simulink model "Network_Standalone"  (R2018b)
settings: Solver=VariableStepAuto  StartTime=0.0  StopTime=10  RelTol=1e-3
undefined symbols (not defined in the file): B, Kd, Ts
libraries: simulink x9
settings Model: Creator=oscar  LastModifiedBy=oscar

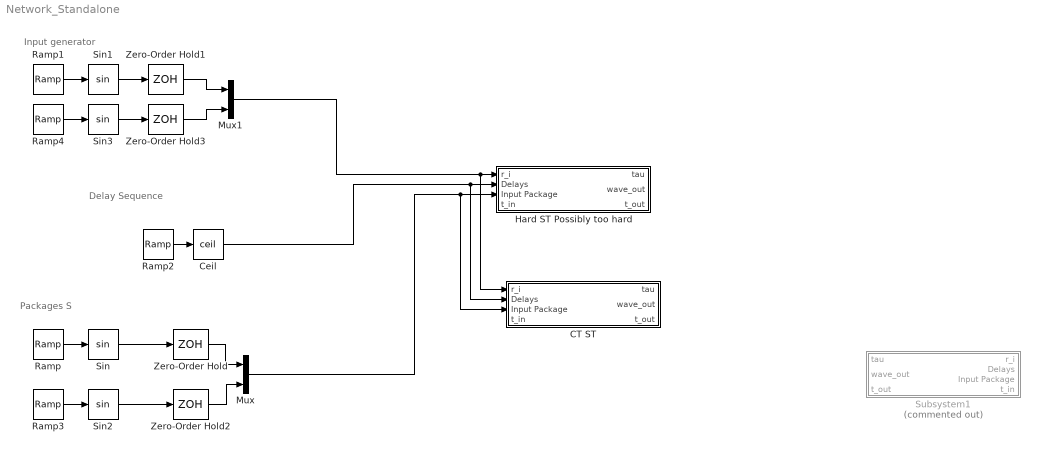
== system Network_Standalone ==
  note: Input generator
  note: Packages S
  note: Delay Sequence
  CT ST : Subsystem
  Ceil : Rounding  Operator=ceil
  Hard ST Possibly too hard : Subsystem
  Mux : Mux  Inputs=2
  Mux1 : Mux  Inputs=2
  Ramp : simulink/Sources/Ramp  slope=1  start=0  InitialOutput=0
  Ramp1 : simulink/Sources/Ramp  slope=1  start=0  InitialOutput=0
  Ramp2 : simulink/Sources/Ramp  slope=0.3/Ts  start=0  InitialOutput=5
  Ramp3 : simulink/Sources/Ramp  slope=0.9  start=1  InitialOutput=0
  Ramp4 : simulink/Sources/Ramp  slope=0.5  start=0  InitialOutput=0
  Sin{,1..3} (4 alike) : Trigonometry
  Subsystem1 : Subsystem  Commented=on
  Zero-Order Hold{,1..3} (4 alike) : ZeroOrderHold  SampleTime=Ts
  wires:
  Ramp/1 -> Sin/1
  Zero-Order Hold/1 -> Mux/1
  Sin/1 -> Zero-Order Hold/1
  Ramp2/1 -> Ceil/1
  Ceil/1 -> CT ST/2(Delays), Hard ST Possibly too hard/2(Delays)
  Zero-Order Hold1/1 -> Mux1/1
  Ramp1/1 -> Sin1/1
  Sin1/1 -> Zero-Order Hold1/1
  Ramp3/1 -> Sin2/1
  Sin2/1 -> Zero-Order Hold2/1
  Mux/1 -> CT ST/3(Input Package), Hard ST Possibly too hard/3(Input Package)
  Zero-Order Hold2/1 -> Mux/2
  Zero-Order Hold3/1 -> Mux1/2
  Mux1/1 -> CT ST/1(r_i), Hard ST Possibly too hard/1(r_i)
  Ramp4/1 -> Sin3/1
  Sin3/1 -> Zero-Order Hold3/1

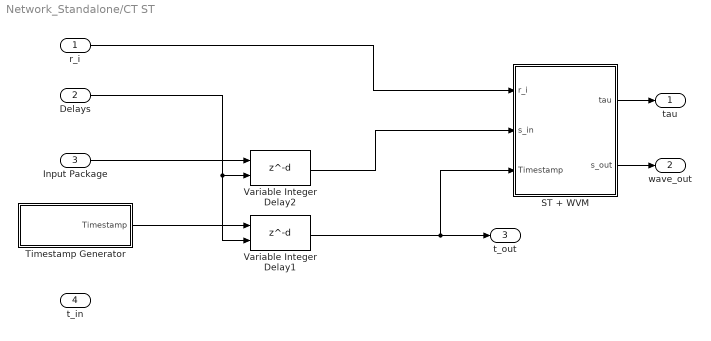
== system Network_Standalone/CT ST ==
  r_i : Inport
  Delays : Inport  Port=2
  Input Package : Inport  Port=3
  t_in : Inport  Port=4
  ST + WVM : Subsystem  TreatAsAtomicUnit=on
  Timestamp Generator : Subsystem
  Variable Integer Delay1 : Delay  DelayLengthSource=Input port  PreventDirectFeedthrough=on  SampleTime=Ts
      settings: InputPortMap=u0,p1
  Variable Integer Delay2 : Delay  DelayLengthSource=Input port  PreventDirectFeedthrough=on  SampleTime=Ts
      settings: InputPortMap=u0,p1
  tau : Outport
  wave_out : Outport  Port=2
  t_out : Outport  Port=3
  wires:
  Input Package/1 -> Variable Integer Delay2/1
  Variable Integer Delay2/1 -> ST + WVM/2(s_in)
  Delays/1 -> Variable Integer Delay1/2, Variable Integer Delay2/2
  Timestamp Generator/1(Timestamp) -> Variable Integer Delay1/1
  r_i/1 -> ST + WVM/1(r_i)
  ST + WVM/1(tau) -> tau/1
  ST + WVM/2(s_out) -> wave_out/1
  Variable Integer Delay1/1 -> ST + WVM/3(Timestamp), t_out/1

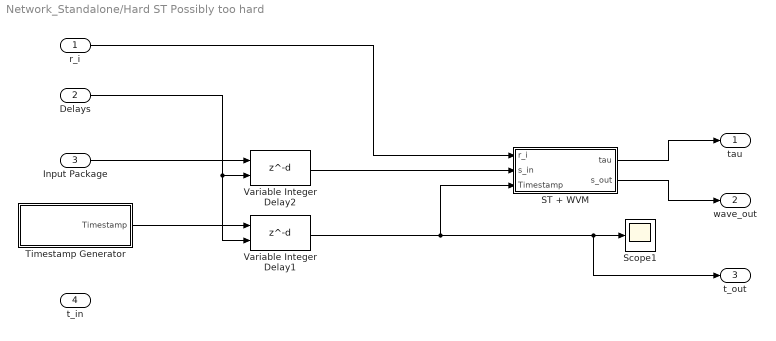
== system Network_Standalone/Hard ST Possibly too hard ==
  r_i : Inport
  Delays : Inport  Port=2
  Input Package : Inport  Port=3
  t_in : Inport  Port=4
  ST + WVM : Subsystem  TreatAsAtomicUnit=on
  Scope1 : Scope
  Timestamp Generator : Subsystem
  Variable Integer Delay1 : Delay  DelayLengthSource=Input port  PreventDirectFeedthrough=on  SampleTime=Ts
      settings: InputPortMap=u0,p1
  Variable Integer Delay2 : Delay  DelayLengthSource=Input port  PreventDirectFeedthrough=on  SampleTime=Ts
      settings: InputPortMap=u0,p1
  tau : Outport
  wave_out : Outport  Port=2
  t_out : Outport  Port=3
  wires:
  Input Package/1 -> Variable Integer Delay2/1
  Variable Integer Delay2/1 -> ST + WVM/2(s_in)
  Delays/1 -> Variable Integer Delay1/2, Variable Integer Delay2/2
  Timestamp Generator/1(Timestamp) -> Variable Integer Delay1/1
  r_i/1 -> ST + WVM/1(r_i)
  ST + WVM/1(tau) -> tau/1
  ST + WVM/2(s_out) -> wave_out/1
  Variable Integer Delay1/1 -> ST + WVM/3(Timestamp), t_out/1, Scope1/1

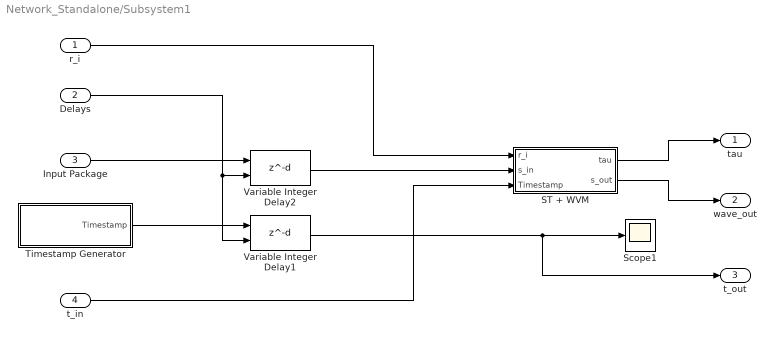
== system Network_Standalone/Subsystem1 ==
  r_i : Inport
  Delays : Inport  Port=2
  Input Package : Inport  Port=3
  t_in : Inport  Port=4
  ST + WVM : Subsystem  TreatAsAtomicUnit=on
  Scope1 : Scope
  Timestamp Generator : Subsystem
  Variable Integer Delay1 : Delay  DelayLengthSource=Input port  PreventDirectFeedthrough=on  SampleTime=Ts
      settings: InputPortMap=u0,p1
  Variable Integer Delay2 : Delay  DelayLengthSource=Input port  PreventDirectFeedthrough=on  SampleTime=Ts
      settings: InputPortMap=u0,p1
  tau : Outport
  wave_out : Outport  Port=2
  t_out : Outport  Port=3
  wires:
  Input Package/1 -> Variable Integer Delay2/1
  Variable Integer Delay2/1 -> ST + WVM/2(s_in)
  Delays/1 -> Variable Integer Delay1/2, Variable Integer Delay2/2
  Timestamp Generator/1(Timestamp) -> Variable Integer Delay1/1
  Variable Integer Delay1/1 -> t_out/1, Scope1/1
  r_i/1 -> ST + WVM/1(r_i)
  ST + WVM/1(tau) -> tau/1
  ST + WVM/2(s_out) -> wave_out/1
  t_in/1 -> ST + WVM/3(Timestamp)

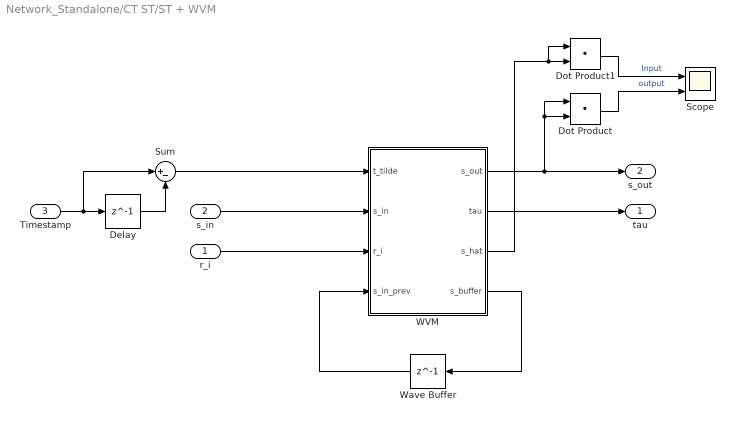
== system Network_Standalone/CT ST/ST + WVM ==
  r_i : Inport
  s_in : Inport  Port=2
  Timestamp : Inport  Port=3
  Delay : Delay  DelayLength=1  SampleTime=Ts
  Dot Product : DotProduct  InputSameDT=on  OutDataTypeStr=Inherit: Inherit via internal rule
  Dot Product1 : DotProduct  InputSameDT=on  OutDataTypeStr=Inherit: Inherit via internal rule
  Scope : Scope  NumInputPorts=2
  Sum : Sum  Inputs=|+-
  WVM : MATLAB Function  TreatAsAtomicUnit=on
  Wave Buffer : Delay  DelayLength=1  InitialCondition=[0;0]  SampleTime=Ts
  tau : Outport
  s_out : Outport  Port=2
  wires:
  Timestamp/1 -> Sum/1, Delay/1
  Delay/1 -> Sum/2
  WVM/2(tau) -> tau/1
  WVM/1(s_out) -> Dot Product/2, Dot Product/1, s_out/1
  WVM/4(s_buffer) -> Wave Buffer/1
  Wave Buffer/1 -> WVM/4(s_in_prev)
  Sum/1 -> WVM/1(t_tilde)
  s_in/1 -> WVM/2(s_in)
  r_i/1 -> WVM/3(r_i)
  WVM/3(s_hat) -> Dot Product1/1, Dot Product1/2
  Dot Product1/1 -> Scope/1  "Input"
  Dot Product/1 -> Scope/2  "output"

== system Network_Standalone/CT ST/Timestamp Generator ==
  note: Timestamp
  Ramp1 : simulink/Sources/Ramp  slope=1/Ts  start=0  InitialOutput=0
  Rounding Function : Rounding
  Timestamp : Outport
  wires:
  Rounding Function/1 -> Timestamp/1
  Ramp1/1 -> Rounding Function/1

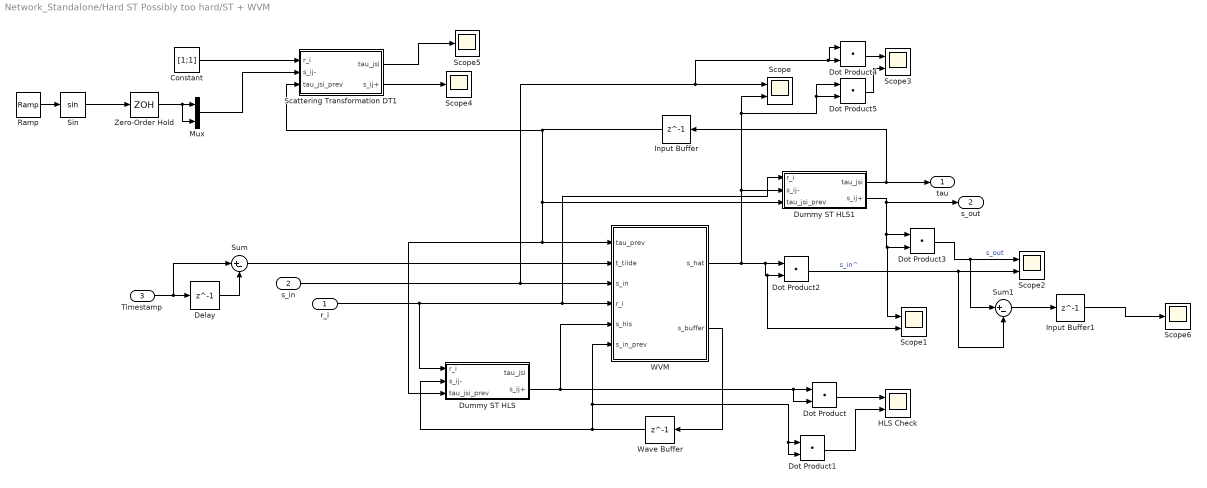
== system Network_Standalone/Hard ST Possibly too hard/ST + WVM ==
  r_i : Inport
  s_in : Inport  Port=2
  Timestamp : Inport  Port=3
  Constant : Constant  Value=[1;1]
  Delay : Delay  DelayLength=1  SampleTime=Ts
  Dot Product{,1..5} (6 alike) : DotProduct  InputSameDT=on  OutDataTypeStr=Inherit: Inherit via internal rule
  Dummy ST HLS : Subsystem
  Dummy ST HLS1 : Subsystem
  HLS Check : Scope  NumInputPorts=2
  Input Buffer : Delay  DelayLength=1  InitialCondition=[0;0]  SampleTime=Ts
  Input Buffer1 : Delay  DelayLength=1  InitialCondition=[0;0]  SampleTime=Ts
  Mux : Mux  Inputs=2
  Ramp : simulink/Sources/Ramp  slope=1  start=0  InitialOutput=0
  Scattering Transformation DT1 : Subsystem
  Scope{,1..3} (4 alike) : Scope  NumInputPorts=2
  Scope4 : Scope
  Scope5 : Scope
  Scope6 : Scope
  Sin : Trigonometry
  Sum : Sum  Inputs=|+-
  Sum1 : Sum  Inputs=|+-
  WVM : MATLAB Function  TreatAsAtomicUnit=on
  Wave Buffer : Delay  DelayLength=1  InitialCondition=[0;0]  SampleTime=Ts
  Zero-Order Hold : ZeroOrderHold  SampleTime=Ts
  tau : Outport
  s_out : Outport  Port=2
  wires:
  Timestamp/1 -> Sum/1, Delay/1
  Delay/1 -> Sum/2
  r_i/1 -> Dummy ST HLS1/1(r_i), WVM/4(r_i), Dummy ST HLS/1(r_i)
  Dummy ST HLS/2(s_ij+) -> Dot Product/2, Dot Product/1, WVM/5(s_hls)
  Dummy ST HLS1/1(tau_jsi) -> Input Buffer/1, tau/1
  Dummy ST HLS1/2(s_ij+) -> Dot Product3/1, Scope1/1, Dot Product3/2, s_out/1
  s_in/1 -> Dot Product4/1, Dot Product4/2, Scope/1, WVM/3(s_in)
  WVM/2(s_buffer) -> Wave Buffer/1
  Sum/1 -> WVM/2(t_tilde)
  Input Buffer/1 -> Scattering Transformation DT1/3(tau_jsi_prev), Dummy ST HLS1/3(tau_jsi_prev), WVM/1(tau_prev), Dummy ST HLS/3(tau_jsi_prev)
  WVM/1(s_hat) -> Scope1/2, Dot Product2/2, Dot Product2/1, Dummy ST HLS1/2(s_ij-), Dot Product5/2, Dot Product5/1, Scope/2
  Dot Product/1 -> HLS Check/1
  Wave Buffer/1 -> Dot Product1/2, Dot Product1/1, WVM/6(s_in_prev), Dummy ST HLS/2(s_ij-)
  Dot Product1/1 -> HLS Check/2
  Dot Product3/1 -> Sum1/1, Scope2/1  "s_out"
  Dot Product4/1 -> Scope3/1
  Dot Product5/1 -> Scope3/2
  Constant/1 -> Scattering Transformation DT1/1(r_i)
  Zero-Order Hold/1 -> Mux/2, Mux/1
  Sin/1 -> Zero-Order Hold/1
  Ramp/1 -> Sin/1
  Scattering Transformation DT1/2(s_ij+) -> Scope4/1
  Scattering Transformation DT1/1(tau_jsi) -> Scope5/1
  Mux/1 -> Scattering Transformation DT1/2(s_ij-)
  Dot Product2/1 -> Sum1/2, Scope2/2  "s_in^"
  Sum1/1 -> Input Buffer1/1
  Input Buffer1/1 -> Scope6/1

== system Network_Standalone/Hard ST Possibly too hard/Timestamp Generator ==
  note: Timestamp
  Ramp1 : simulink/Sources/Ramp  slope=1/Ts  start=0  InitialOutput=0
  Rounding Function : Rounding
  Timestamp : Outport
  wires:
  Rounding Function/1 -> Timestamp/1
  Ramp1/1 -> Rounding Function/1

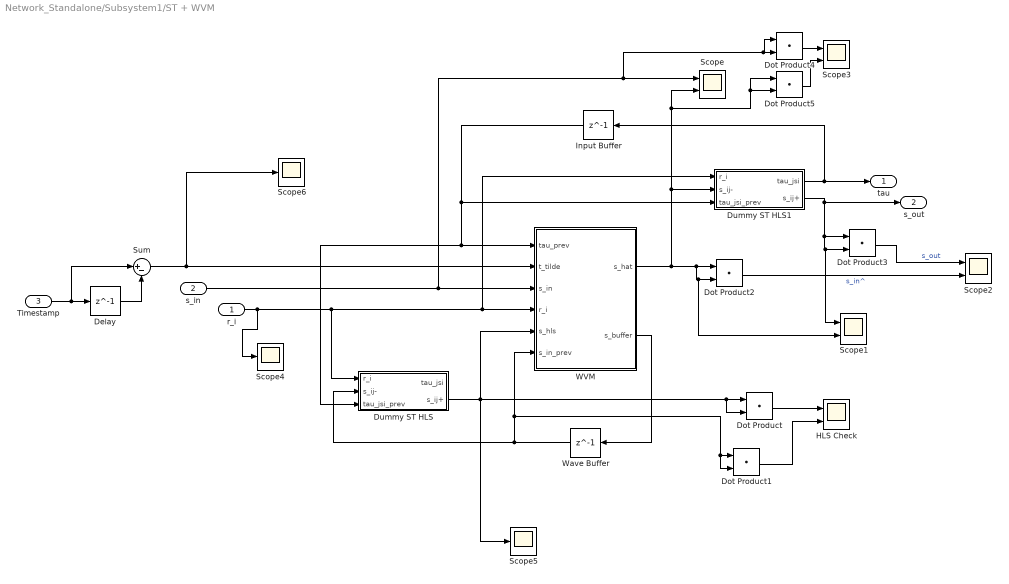
== system Network_Standalone/Subsystem1/ST + WVM ==
  r_i : Inport
  s_in : Inport  Port=2
  Timestamp : Inport  Port=3
  Delay : Delay  DelayLength=1  SampleTime=Ts
  Dot Product{,1..5} (6 alike) : DotProduct  InputSameDT=on  OutDataTypeStr=Inherit: Inherit via internal rule
  Dummy ST HLS : Subsystem
  Dummy ST HLS1 : Subsystem
  HLS Check : Scope  NumInputPorts=2
  Input Buffer : Delay  DelayLength=1  InitialCondition=[0;0]  SampleTime=Ts
  Scope{,1..3} (4 alike) : Scope  NumInputPorts=2
  Scope4 : Scope
  Scope5 : Scope
  Scope6 : Scope
  Sum : Sum  Inputs=|+-
  WVM : MATLAB Function  TreatAsAtomicUnit=on
  Wave Buffer : Delay  DelayLength=1  InitialCondition=[0;0]  SampleTime=Ts
  tau : Outport
  s_out : Outport  Port=2
  wires:
  Timestamp/1 -> Sum/1, Delay/1
  Delay/1 -> Sum/2
  r_i/1 -> Scope4/1, Dummy ST HLS1/1(r_i), WVM/4(r_i), Dummy ST HLS/1(r_i)
  Dummy ST HLS/2(s_ij+) -> Scope5/1, Dot Product/2, Dot Product/1, WVM/5(s_hls)
  Dummy ST HLS1/1(tau_jsi) -> Input Buffer/1, tau/1
  Dummy ST HLS1/2(s_ij+) -> Dot Product3/1, Scope1/1, Dot Product3/2, s_out/1
  s_in/1 -> Dot Product4/1, Dot Product4/2, Scope/1, WVM/3(s_in)
  WVM/2(s_buffer) -> Wave Buffer/1
  Sum/1 -> Scope6/1, WVM/2(t_tilde)
  Input Buffer/1 -> Dummy ST HLS1/3(tau_jsi_prev), WVM/1(tau_prev), Dummy ST HLS/3(tau_jsi_prev)
  WVM/1(s_hat) -> Scope1/2, Dot Product2/2, Dot Product2/1, Dummy ST HLS1/2(s_ij-), Dot Product5/2, Dot Product5/1, Scope/2
  Dot Product/1 -> HLS Check/1
  Wave Buffer/1 -> Dot Product1/2, Dot Product1/1, WVM/6(s_in_prev), Dummy ST HLS/2(s_ij-)
  Dot Product1/1 -> HLS Check/2
  Dot Product3/1 -> Scope2/1  "s_out"
  Dot Product4/1 -> Scope3/1
  Dot Product5/1 -> Scope3/2
  Dot Product2/1 -> Scope2/2  "s_in^"

== system Network_Standalone/Subsystem1/Timestamp Generator ==
  note: Timestamp
  Ramp1 : simulink/Sources/Ramp  slope=1/Ts  start=0  InitialOutput=0
  Rounding Function : Rounding
  Timestamp : Outport
  wires:
  Rounding Function/1 -> Timestamp/1
  Ramp1/1 -> Rounding Function/1

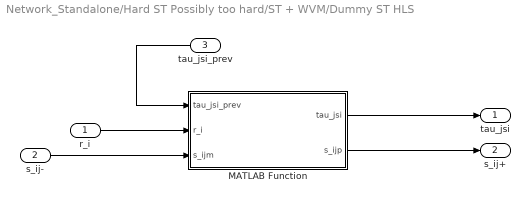
== system Network_Standalone/Hard ST Possibly too hard/ST + WVM/Dummy ST HLS ==
  r_i : Inport
  s_ij- : Inport  Port=2
  tau_jsi_prev : Inport  Port=3
  MATLAB Function : MATLAB Function  TreatAsAtomicUnit=on
  tau_jsi : Outport
  s_ij+ : Outport  Port=2
  wires:
  MATLAB Function/1(tau_jsi) -> tau_jsi/1
  tau_jsi_prev/1 -> MATLAB Function/1(tau_jsi_prev)
  r_i/1 -> MATLAB Function/2(r_i)
  s_ij-/1 -> MATLAB Function/3(s_ijm)
  MATLAB Function/2(s_ijp) -> s_ij+/1

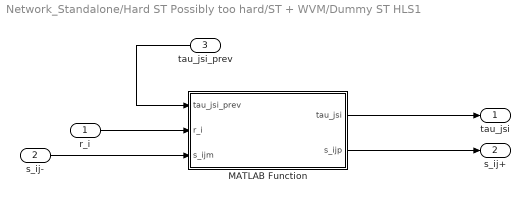
== system Network_Standalone/Hard ST Possibly too hard/ST + WVM/Dummy ST HLS1 ==
  r_i : Inport
  s_ij- : Inport  Port=2
  tau_jsi_prev : Inport  Port=3
  MATLAB Function : MATLAB Function  TreatAsAtomicUnit=on
  tau_jsi : Outport
  s_ij+ : Outport  Port=2
  wires:
  MATLAB Function/1(tau_jsi) -> tau_jsi/1
  tau_jsi_prev/1 -> MATLAB Function/1(tau_jsi_prev)
  r_i/1 -> MATLAB Function/2(r_i)
  s_ij-/1 -> MATLAB Function/3(s_ijm)
  MATLAB Function/2(s_ijp) -> s_ij+/1

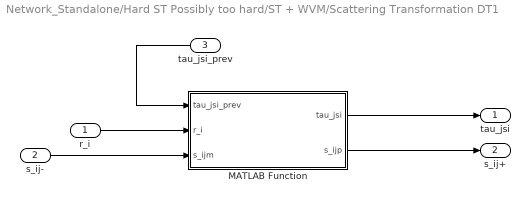
== system Network_Standalone/Hard ST Possibly too hard/ST + WVM/Scattering Transformation DT1 ==
  r_i : Inport
  s_ij- : Inport  Port=2
  tau_jsi_prev : Inport  Port=3
  MATLAB Function : MATLAB Function  TreatAsAtomicUnit=on
  tau_jsi : Outport
  s_ij+ : Outport  Port=2
  wires:
  MATLAB Function/1(tau_jsi) -> tau_jsi/1
  tau_jsi_prev/1 -> MATLAB Function/1(tau_jsi_prev)
  r_i/1 -> MATLAB Function/2(r_i)
  s_ij-/1 -> MATLAB Function/3(s_ijm)
  MATLAB Function/2(s_ijp) -> s_ij+/1

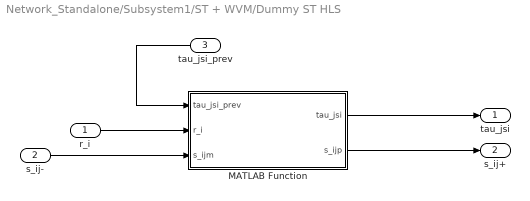
== system Network_Standalone/Subsystem1/ST + WVM/Dummy ST HLS ==
  r_i : Inport
  s_ij- : Inport  Port=2
  tau_jsi_prev : Inport  Port=3
  MATLAB Function : MATLAB Function  TreatAsAtomicUnit=on
  tau_jsi : Outport
  s_ij+ : Outport  Port=2
  wires:
  MATLAB Function/1(tau_jsi) -> tau_jsi/1
  tau_jsi_prev/1 -> MATLAB Function/1(tau_jsi_prev)
  r_i/1 -> MATLAB Function/2(r_i)
  s_ij-/1 -> MATLAB Function/3(s_ijm)
  MATLAB Function/2(s_ijp) -> s_ij+/1

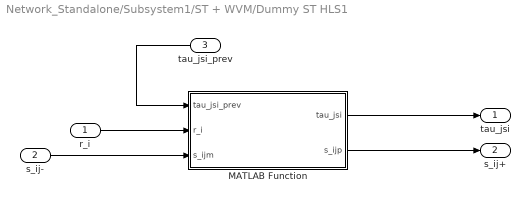
== system Network_Standalone/Subsystem1/ST + WVM/Dummy ST HLS1 ==
  r_i : Inport
  s_ij- : Inport  Port=2
  tau_jsi_prev : Inport  Port=3
  MATLAB Function : MATLAB Function  TreatAsAtomicUnit=on
  tau_jsi : Outport
  s_ij+ : Outport  Port=2
  wires:
  MATLAB Function/1(tau_jsi) -> tau_jsi/1
  tau_jsi_prev/1 -> MATLAB Function/1(tau_jsi_prev)
  r_i/1 -> MATLAB Function/2(r_i)
  s_ij-/1 -> MATLAB Function/3(s_ijm)
  MATLAB Function/2(s_ijp) -> s_ij+/1

== matlab function Network_Standalone/Hard ST Possibly too hard/ST + WVM/Scattering Transformation DT1/MATLAB Function ==
  data: tau_jsi_prev input; r_i input; tau_jsi output; s_ijm input; s_ijp output; B parameter; Kd parameter
function [tau_jsi, s_ijp] = STL(tau_jsi_prev,r_i, s_ijm, B, Kd)
    tau_jsi = zeros(2, 1);
    s_ijp = zeros(2, 1);
    
    r_js = (inv(B))^2*(-sqrt(2)*B*s_ijm - tau_jsi_prev);
    tau_jsi = Kd*(r_js - r_i);
    s_ijp = 1/sqrt(2)*inv(B)*(-tau_jsi + B^2*r_js);
end

== matlab function Network_Standalone/Hard ST Possibly too hard/ST + WVM/Dummy ST HLS1/MATLAB Function ==
  data: tau_jsi_prev input; r_i input; tau_jsi output; s_ijm input; s_ijp output; B parameter; Kd parameter
function [tau_jsi, s_ijp] = STL(tau_jsi_prev,r_i, s_ijm, B, Kd)
    tau_jsi = zeros(2, 1);
    s_ijp = zeros(2, 1);
    
    r_js = (inv(B))^2*(-sqrt(2)*B*s_ijm - tau_jsi_prev);
    tau_jsi = Kd*(r_js - r_i);
    s_ijp = 1/sqrt(2)*inv(B)*(-tau_jsi_prev + B^2*r_js);
end

== matlab function Network_Standalone/Hard ST Possibly too hard/ST + WVM/WVM ==
  data: tau_prev input; t_tilde input; s_in input; r_i input; s_hls input; s_in_prev input; s_hat output; s_buffer output
function [s_hat, s_buffer]  = fcn(tau_prev, t_tilde, s_in, r_i, s_hls, s_in_prev)
    s_hat = zeros(2, 1);
    s_buffer = zeros(2, 1);
    
    %% If 0 then no new data -> reconstruct!
    % If lower than 0, then the package is reordered and we reject the
    % package
    if(t_tilde <= 0)  
        % If HLS is passive apply HLS
        if(s_hls'*s_hls >= s_in_prev'*s_in_prev)
            s_hat = s_in_prev;
            
        % Otherwise apply the acceptable magnitude in that direction
        else
            s_hat = zeros(2,1);%sign(s_in_prev).*abs(s_hls)./sqrt(2);
            %s_hat = sign(s_in_prev) .* abs(1/sqrt(2)*r_i); % WVM Gain (Dit is nie netjes)
        end
        
        % Either way repeat the last value
        s_buffer = s_in_prev;
        
    %% If 1 then no weird shenanigans, data arrived on time
    %% If > 1 then the packages are reordered and we keep the last one
    else
        s_hat = s_in; % Use the received value
        s_buffer = s_in; % And store its value
    end    

end

== matlab function Network_Standalone/Hard ST Possibly too hard/ST + WVM/Dummy ST HLS/MATLAB Function ==
  data: tau_jsi_prev input; r_i input; tau_jsi output; s_ijm input; s_ijp output; B parameter; Kd parameter
function [tau_jsi, s_ijp] = STL(tau_jsi_prev,r_i, s_ijm, B, Kd)
    tau_jsi = zeros(2, 1);
    s_ijp = zeros(2, 1);
    
    r_js = (inv(B))^2*(-sqrt(2)*B*s_ijm - tau_jsi_prev);
    tau_jsi = Kd*(r_js - r_i);
    s_ijp = 1/sqrt(2)*inv(B)*(-tau_jsi_prev + B^2*r_js);
end

== matlab function Network_Standalone/Subsystem1/ST + WVM/Dummy ST HLS/MATLAB Function ==
  data: tau_jsi_prev input; r_i input; tau_jsi output; s_ijm input; s_ijp output; B parameter; Kd parameter
function [tau_jsi, s_ijp] = STL(tau_jsi_prev,r_i, s_ijm, B, Kd)
    tau_jsi = zeros(2, 1);
    s_ijp = zeros(2, 1);
    
    r_js = (inv(B))^2*(sqrt(2)*B*s_ijm - tau_jsi_prev);
    tau_jsi = Kd*(r_js - r_i);
    s_ijp = 1/sqrt(2)*inv(B)*(tau_jsi - B^2*r_js);
end

== matlab function Network_Standalone/Subsystem1/ST + WVM/Dummy ST HLS1/MATLAB Function ==
  data: tau_jsi_prev input; r_i input; tau_jsi output; s_ijm input; s_ijp output; B parameter; Kd parameter
function [tau_jsi, s_ijp] = STL(tau_jsi_prev,r_i, s_ijm, B, Kd)
    tau_jsi = zeros(2, 1);
    s_ijp = zeros(2, 1);
    
    r_js = (inv(B))^2*(sqrt(2)*B*s_ijm - tau_jsi_prev);
    tau_jsi = Kd*(r_js - r_i);
    s_ijp = 1/sqrt(2)*inv(B)*(tau_jsi - B^2*r_js);
end

== matlab function Network_Standalone/Subsystem1/ST + WVM/WVM ==
  data: tau_prev input; t_tilde input; s_in input; r_i input; s_hls input; s_in_prev input; s_hat output; s_buffer output
function [s_hat, s_buffer]  = fcn(tau_prev, t_tilde, s_in, r_i, s_hls, s_in_prev)
    s_hat = zeros(2, 1);
    s_buffer = zeros(2, 1);
    
    %% If 0 then no new data -> reconstruct!
    % If lower than 0, then the package is reordered and we reject the
    % package
    if(t_tilde <= 0)  
        % If HLS is passive apply HLS
        if(s_hls'*s_hls >= s_in_prev'*s_in_prev)
            s_hat = s_in_prev;
            
        % Otherwise apply the acceptable magnitude in that direction
        else
            s_hat = zeros(2,1);%sign(s_in_prev).*abs(s_hls)./sqrt(2);
            %s_hat = sign(s_in_prev) .* abs(1/sqrt(2)*r_i); % WVM Gain (Dit is nie netjes)
        end
        
        % Either way repeat the last value
        s_buffer = s_in_prev;
        
    %% If 1 then no weird shenanigans, data arrived on time
    %% If > 1 then the packages are reordered and we keep the last one
    else
        s_hat = s_in; % Use the received value
        s_buffer = s_in; % And store its value
    end    

end

== matlab function Network_Standalone/CT ST/ST + WVM/WVM ==
  data: t_tilde input; s_in input; r_i input; s_in_prev input; s_out output; tau output; s_hat output; s_buffer output; KL parameter
function [s_out, tau, s_hat, s_buffer]  = fcn(t_tilde, s_in, r_i, s_in_prev, KL)
    s_hat = zeros(2, 1);
    s_buffer = zeros(2, 1);
    s_out = zeros(2, 1);
    tau = zeros(2, 1);
    
    %% If 0 then no new data -> reconstruct!
    % If lower than 0, then the package is reordered and we reject the
    % package
    if(t_tilde <= 0)  
        % WVM
        Y = KL*[s_in_prev; r_i];
        s_hls = Y(3:4);
        
        % If HLS is passive apply HLS
        if(s_hls'*s_hls >= s_in_prev'*s_in_prev)
            s_hat = s_in_prev;
            
        % Otherwise apply the acceptable magnitude in that direction
        else
            s_hat = sign(s_in_prev).*abs(s_hls);
        end
        
        % Either way repeat the last value
        s_buffer = s_in_prev;
        
    %% If 1 then no weird shenanigans, data arrived on time
    %% If > 1 then the packages are reordered and we keep the last one
    else
        s_hat = s_in; % Use the received value
        s_buffer = s_in; % And store its value
    end    
    
    Y = KL*[s_hat; r_i];
    tau = Y(1:2); s_out = Y(3:4);

end
